simulink model "sampleModel212"  (R2021b)
settings: Solver=VariableStepAuto  StartTime=0.0  StopTime=10.0  RelTol=1e-3
undefined symbols (not defined in the file or in its folder): DiscIntNeverNeededParam, Newton, Raphson
libraries: simulink x6, slpidlib x1
settings Model: Creator=user  LastModifiedBy=user

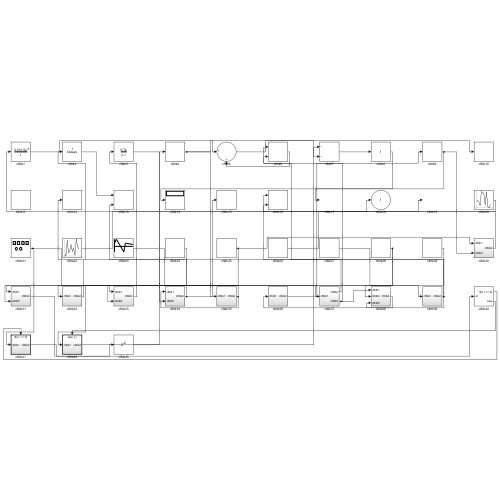
[thumbnail: Simulink's stored preview of the top-level diagram]
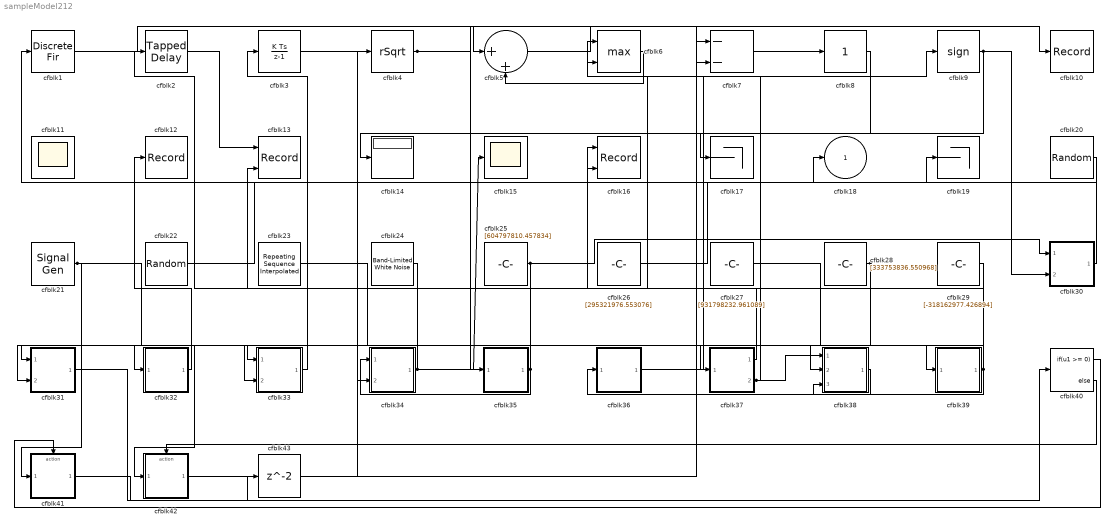
== system sampleModel212 ==
  cfblk1 : DiscreteFir  SampleTime=1
  cfblk10 : Record  FileSettingsInternal="{\"entries\":[{\"content\":{\"excelSettings\":{\"content\":{},\"type\":\"Streamout.ExcelSettings\"}},\"type\":\"Streamout.FileSettingStorage\",\"uuid\":\"9136f186-ec9e-49fd-8053-90c4ae60cd6f\"}],\"packageUris\":[\"http://schema.mathworks.com/mf0/streamout_blocks/R2020a\"],\"version\":\"1.0\"}"  SignalsInternal="{\"entries\":[{\"content\":{\"signals\":[{\"content\":{\"blockPath\":[\"sampleModel212/cfblk10\"],\"channel\":[],\"dimensions\":[1],\"domain\":\"sampleModel212/cfblk10\",\"lineColor\":\"#edb120\",\"plots\":[1],\"port\":1,\"sid\":[\"\"],\"signalID\":8232,\"signalName\":\"cfblk5\"},\"type\":\"RecordBlkView.Signal\",\"uuid\":\"3d6c6ed9-3216-4515-a2b3-ec71c8580300\"}]},\"type\":\"RecordBlkView.InputSignals\",\"uuid\":\"6f53bf0b-d229-4304-8eb9-cf2f8789923b\"}],\"packageUris\":[\"http://schema.mathworks.com/mf0/streamout_blocks/R2020a\"],\"version\":\"1.0\"}"  VisualizationBindings="{\"sparklinesplugin\":{\"info\":[{\"bindingParametersList\":[],\"subplotID\":1}]}}"
  cfblk11 : Scope
      settings: Floating=on
  cfblk12 : Record  FileSettingsInternal="{\"entries\":[{\"content\":{\"excelSettings\":{\"content\":{},\"type\":\"Streamout.ExcelSettings\"}},\"type\":\"Streamout.FileSettingStorage\",\"uuid\":\"6ba16359-3d74-4ac6-a319-7b95d1bddcf9\"}],\"packageUris\":[\"http://schema.mathworks.com/mf0/streamout_blocks/R2020a\"],\"version\":\"1.0\"}"  SignalsInternal="{\"entries\":[{\"content\":{\"signals\":[{\"content\":{\"blockPath\":[\"sampleModel212/cfblk12\"],\"channel\":[],\"dimensions\":[1],\"domain\":\"sampleModel212/cfblk12\",\"lineColor\":\"#139fff\",\"plots\":[1],\"port\":1,\"sid\":[\"\"],\"signalID\":8252,\"signalName\":\"cfblk32\"},\"type\":\"RecordBlkView.Signal\",\"uuid\":\"2d56ea30-9116-46ed-9e82-5e82888dbfa9\"}]},\"type\":\"RecordBlkView.InputSignals\",\"uuid\":\"56d7414f-cbe6-4e07-9f56-36ce9f4febc1\"}],\"packageUris\":[\"http://schema.mathworks.com/mf0/streamout_blocks/R2020a\"],\"version\":\"1.0\"}"  VisualizationBindings="{\"sparklinesplugin\":{\"info\":[{\"bindingParametersList\":[],\"subplotID\":1}]}}"
  cfblk13 : Record  FileSettingsInternal="{\"entries\":[{\"content\":{\"excelSettings\":{\"content\":{},\"type\":\"Streamout.ExcelSettings\"}},\"type\":\"Streamout.FileSettingStorage\",\"uuid\":\"0acae2d6-ee60-4856-b366-a0806cd00a70\"}],\"packageUris\":[\"http://schema.mathworks.com/mf0/streamout_blocks/R2020a\"],\"version\":\"1.0\"}"  Layout=[1 1]  SignalsInternal="{\"entries\":[{\"content\":{\"signals\":[{\"content\":{\"blockPath\":[\"sampleModel212/cfblk13\"],\"channel\":[],\"dimensions\":[1],\"domain\":\"sampleModel212/cfblk13\",\"lineColor\":\"#a2142f\",\"plots\":[1],\"port\":1,\"sid\":[\"\"],\"signalID\":8236,\"signalName\":\"cfblk2\"},\"type\":\"RecordBlkView.Signal\",\"uuid\":\"529bd515-27fc-4e1a-94ea-2d07532aa9c1\"},{\"content\":{\"blockPath\":[\"sampleModel212/cfblk13\"],\"channel\":[],\"dimensions\":[1],\"domain\":\"sampleModel212/cfblk13\",\"lineColor\":\"#139fff\",\"plots\":[1],\"port\":2,\"sid\":[\"\"],\"signalID\":8240,\"signalName\":\"cfblk39\"},\"type\":\"RecordBlkView.Signal\",\"uuid\":\"26540efe-244b-4170-a373-6d34e17a1cae\"}]},\"type\":\"RecordBlkView.InputSignals\",\"uuid\":\"31d81cea-1ae4-4f42-aa9f-f175325ecb32\"}],\"packageUris\":[\"http://schema.mathworks.com/mf0/streamout_blocks/R2020a\"],\"version\":\"1.0\"}"  VisualizationBindings="{\"xyplotplugin\":{\"info\":[{\"series\":[{\"bindingParametersList\":[{\"parameter\":\"X-Axis\",\"signalID\":8236,\"signalName\":\"cfblk2\"},{\"parameter\":\"Y-Axis\",\"signalID\":8240,\"signalName\":\"cfblk39\"}],\"seriesID\":42465}],\"subplotID\":1}]}}"  CompatibilityTag=XY
  cfblk14 : Display
  cfblk15 : Scope
  cfblk16 : Record  FileSettingsInternal="{\"entries\":[{\"content\":{\"excelSettings\":{\"content\":{},\"type\":\"Streamout.ExcelSettings\"}},\"type\":\"Streamout.FileSettingStorage\",\"uuid\":\"ca503a4a-a96d-43a1-9ebc-70d0128dd941\"}],\"packageUris\":[\"http://schema.mathworks.com/mf0/streamout_blocks/R2020a\"],\"version\":\"1.0\"}"  Layout=[1 1]  SignalsInternal="{\"entries\":[{\"content\":{\"signals\":[{\"content\":{\"blockPath\":[\"sampleModel212/cfblk16\"],\"channel\":[],\"dimensions\":[1],\"domain\":\"sampleModel212/cfblk16\",\"lineColor\":\"#a2142f\",\"plots\":[1],\"port\":1,\"sid\":[\"\"],\"signalID\":8244,\"signalName\":\"cfblk37:1\"},\"type\":\"RecordBlkView.Signal\",\"uuid\":\"e63eec24-58ba-4f65-805e-17e2aa971a90\"},{\"content\":{\"blockPath\":[\"sampleModel212/cfblk16\"],\"channel\":[],\"dimensions\":[1],\"domain\":\"sampleModel212/cfblk16\",\"lineColor\":\"#139fff\",\"plots\":[1],\"port\":2,\"sid\":[\"\"],\"signalID\":8248,\"signalName\":\"cfblk20\"},\"type\":\"RecordBlkView.Signal\",\"uuid\":\"84022ab3-d0b3-46d1-9cc4-89043ad64550\"}]},\"type\":\"RecordBlkView.InputSignals\",\"uuid\":\"213b04ee-a0f2-43b0-a9ef-411359d2bb67\"}],\"packageUris\":[\"http://schema.mathworks.com/mf0/streamout_blocks/R2020a\"],\"version\":\"1.0\"}"  VisualizationBindings="{\"xyplotplugin\":{\"info\":[{\"series\":[{\"bindingParametersList\":[{\"parameter\":\"X-Axis\",\"signalID\":8244,\"signalName\":\"cfblk37:1\"},{\"parameter\":\"Y-Axis\",\"signalID\":8248,\"signalName\":\"cfblk20\"}],\"seriesID\":43597}],\"subplotID\":1}]}}"  CompatibilityTag=XY
  cfblk17 : Terminator
  cfblk19 : Terminator
  cfblk2 : simulink/Discrete/Tapped Delay  vinit=0.0  samptime=-1  NumDelays=1  DelayOrder=Oldest  includeCurrent=off
  cfblk20 : RandomNumber  Mean=[74771.324273]  Variance=[43680.592014]  Seed=[211738287.000000]  SampleTime=0.1
  cfblk21 : SignalGenerator  WaveForm=square  Amplitude=[-349925656.261152]
  cfblk22 : UniformRandomNumber  Minimum=[-1543428115.464297]  Maximum=[1225243770.020049]  Seed=[69964703.000000]  SampleTime=0.1
  cfblk23 : simulink/Sources/Repeating Sequence Interpolated  OutValues=[224382166.710449, 496779107.925151, -364574655.609755, 227281435.577570, 132134347.634255]  TimeValues=[0 0.1 0.5 0.6 1].'  LookUpMeth=Use Input Below  tsamp=0.01  OutMin=[]  OutMax=[]  OutDataTypeStr=double  OutputDataTypeScalingMode=double  OutDataType=fixdt(0,8)  OutScaling=2^-10
  cfblk24 : simulink/Sources/Band-Limited White Noise  Cov=[1404469097.228225]  Ts=0.1  seed=[6451413531.000000]
  cfblk25 : Constant  Value=[604797810.457834]  SampleTime=1
  cfblk26 : Constant  Value=[295321976.553076]  SampleTime=1
  cfblk27 : Constant  Value=[931798232.961089]  SampleTime=1
  cfblk28 : Constant  Value=[333753836.550968]  SampleTime=1
  cfblk29 : Constant  Value=[-318162977.426894]  SampleTime=1
  cfblk3 : DiscreteIntegrator  ICPrevOutput=DiscIntNeverNeededParam  ICPrevScaledInput=DiscIntNeverNeededParam
  cfblk30 : Subsystem
  cfblk31 : Subsystem
  cfblk32 : Subsystem
  cfblk33 : Subsystem
  cfblk34 : Subsystem
  cfblk35 : Subsystem
  cfblk36 : Subsystem
  cfblk37 : Subsystem
  cfblk38 : Subsystem
  cfblk39 : Subsystem
  cfblk4 : Sqrt  Operator=rSqrt  AlgorithmType=Newton-Raphson  SaturateOnIntegerOverflow=on
  cfblk40 : If  IfExpression=u1 >= 0  SampleTime=1
  cfblk41 : Subsystem  TreatAsAtomicUnit=on
  cfblk42 : Subsystem  TreatAsAtomicUnit=on
  cfblk43 : Delay  SampleTime=1
  cfblk5 : Sum  Inputs=|++
  cfblk6 : MinMax  Function=max  Inputs=2
  cfblk7 : Sum  Inputs=--
  cfblk8 : simulink/Math Operations/Slider Gain  gain=1  low=0  high=2
  cfblk9 : Signum
  cfblk18 : Outport
  wires:
  cfblk30/1(cfblk2) -> cfblk1/1
  cfblk7/1 -> cfblk8/1
  cfblk29/1 -> cfblk32/1(cfblk1)
  cfblk2/1 -> cfblk13/1
  cfblk34/1(cfblk2) -> cfblk15/1, cfblk2/1
  cfblk32/1(cfblk2) -> cfblk12/1
  cfblk4/1 -> cfblk35/1(cfblk1), cfblk7/2
  cfblk33/1(cfblk2) -> cfblk3/1
  cfblk35/1(cfblk2) -> cfblk34/1(cfblk1), cfblk31/1(cfblk1)
  cfblk25/1 -> cfblk33/1(cfblk1), cfblk30/1(cfblk1)
  cfblk36/1(cfblk2) -> cfblk9/1
  cfblk38/1(cfblk2) -> cfblk36/1(cfblk1)
  cfblk1/1 -> cfblk5/1
  cfblk23/1 -> cfblk37/1(cfblk1)
  cfblk42/1(cfblk2) -> cfblk7/1
  cfblk39/1(cfblk2) -> cfblk13/2, cfblk38/3(cfblk5), cfblk6/1
  cfblk24/1 -> cfblk42/1(cfblk1)
  cfblk21/1 -> cfblk33/2(cfblk4), cfblk41/1(cfblk1)
  cfblk6/1 -> cfblk5/2
  cfblk8/1 -> cfblk14/1
  cfblk37/1(cfblk2) -> cfblk16/1
  cfblk27/1 -> cfblk39/1(cfblk1)
  cfblk22/1 -> cfblk18/1
  cfblk37/2(cfblk3) -> cfblk38/1(cfblk1), cfblk6/2
  cfblk20/1 -> cfblk16/2
  cfblk3/1 -> cfblk34/2(cfblk5)
  cfblk9/1 -> cfblk17/1, cfblk30/2(cfblk5)
  cfblk26/1 -> cfblk19/1
  cfblk28/1 -> cfblk38/2(cfblk4), cfblk31/2(cfblk5)
  cfblk31/1(cfblk2) -> cfblk40/1
  cfblk5/1 -> cfblk10/1
  cfblk40/1 -> cfblk41/Action
  cfblk40/2 -> cfblk42/Action
  cfblk41/1(cfblk2) -> cfblk43/1
  cfblk43/1 -> cfblk4/1

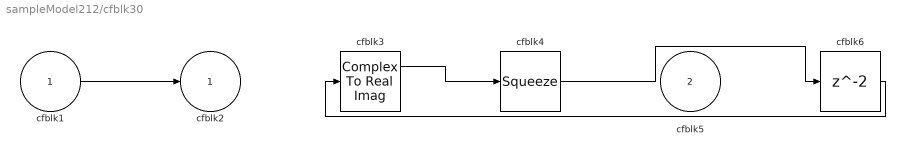
== system sampleModel212/cfblk30 ==
  cfblk1 : Inport
  cfblk5 : Inport  Port=2
  cfblk3 : ComplexToRealImag
  cfblk4 : Squeeze
  cfblk6 : Delay  SampleTime=1
  cfblk2 : Outport
  wires:
  cfblk1/1 -> cfblk2/1
  cfblk3/1 -> cfblk4/1
  cfblk4/1 -> cfblk6/1
  cfblk6/1 -> cfblk3/1

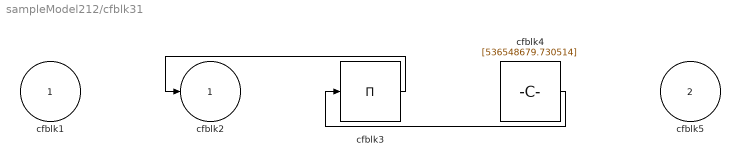
== system sampleModel212/cfblk31 ==
  cfblk1 : Inport
  cfblk5 : Inport  Port=2
  cfblk3 : Product  Inputs=*
  cfblk4 : Constant  Value=[536548679.730514]  SampleTime=1
  cfblk2 : Outport
  wires:
  cfblk3/1 -> cfblk2/1
  cfblk4/1 -> cfblk3/1

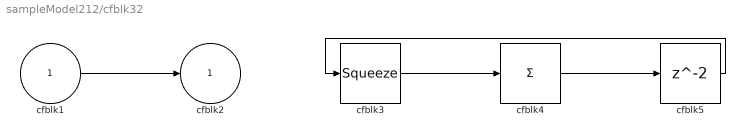
== system sampleModel212/cfblk32 ==
  cfblk1 : Inport
  cfblk3 : Squeeze
  cfblk4 : Sum  Inputs=+
  cfblk5 : Delay  SampleTime=1
  cfblk2 : Outport
  wires:
  cfblk3/1 -> cfblk4/1
  cfblk1/1 -> cfblk2/1
  cfblk4/1 -> cfblk5/1
  cfblk5/1 -> cfblk3/1

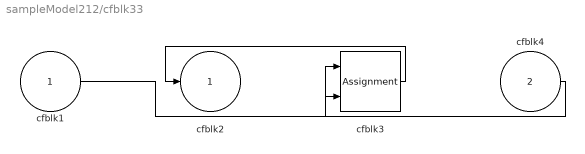
== system sampleModel212/cfblk33 ==
  cfblk1 : Inport
  cfblk4 : Inport  Port=2
  cfblk3 : Assignment  DiagnosticForDimensions=Warning  IndexOptions=Index vector (dialog)  Indices=1  OutputSizes=1
  cfblk2 : Outport
  wires:
  cfblk3/1 -> cfblk2/1
  cfblk1/1 -> cfblk3/1
  cfblk4/1 -> cfblk3/2

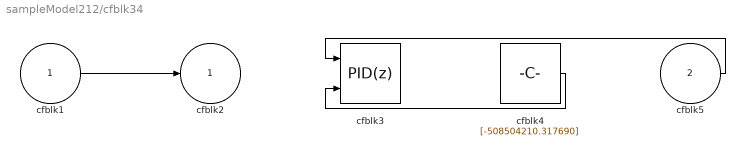
== system sampleModel212/cfblk34 ==
  cfblk1 : Inport
  cfblk5 : Inport  Port=2
  cfblk3 : slpidlib/PID Controller (2DOF)  Controller=PID  Form=Parallel  TimeDomain=Discrete-time  UseExternalTs=off  SampleTime=1  IntegratorMethod=Forward Euler  FilterMethod=Forward Euler  ControllerParametersSource=internal  P=1  I=1  D=0  UseFilter=on  N=100  b=1  c=1  TunerSelectOption=Transfer Function Based (PID Tuner App)  InitialConditionSource=internal  InitialConditionForIntegrator=0  InitialConditionForFilter=0  DifferentiatorICPrevScaledInput=0  ExternalReset=none  TrackingMode=off  Kt=1  LimitOutput=off  SatLimitsSource=internal  UpperSaturationLimit=inf  LowerSaturationLimit=-inf  LinearizeAsGain=off  AntiWindupMode=none  Kb=1  POutMin=[]  POutMax=[]  IOutMin=[]  IOutMax=[]  DOutMin=[]  DOutMax=[]  NOutMin=[]  NOutMax=[]  bOutMin=[]  bOutMax=[]  cOutMin=[]  cOutMax=[]  SumOutMin=[]  SumOutMax=[]  SaturationOutMin=[]  SaturationOutMax=[]  PParamMin=[]  PParamMax=[]  IParamMin=[]  IParamMax=[]  DParamMin=[]  DParamMax=[]  NParamMin=[]  NParamMax=[]  bParamMin=[]  bParamMax=[]  cParamMin=[]  cParamMax=[]  KbParamMin=[]  KbParamMax=[]  KtParamMin=[]  KtParamMax=[]  KbOutMin=[]  KbOutMax=[]  KtOutMin=[]  KtOutMax=[]  IntegratorOutMin=[]  IntegratorOutMax=[]  FilterOutMin=[]  FilterOutMax=[]  SumI1OutMin=[]  SumI1OutMax=[]  SumI2OutMin=[]  SumI2OutMax=[]  SumI3OutMin=[]  SumI3OutMax=[]  SumI4OutMin=[]  SumI4OutMax=[]  SumDOutMin=[]  SumDOutMax=[]  Sum1OutMin=[]  Sum1OutMax=[]  Sum2OutMin=[]  Sum2OutMax=[]  Sum3OutMin=[]  Sum3OutMax=[]  DifferentiatorOutMin=[]  DifferentiatorOutMax=[]  FilterDiffOutCoefMin=[]  FilterDiffOutCoefMax=[]  ReciprocalOutMin=[]  ReciprocalOutMax=[]  SumDenOutMin=[]  SumDenOutMax=[]  SumNumOutMin=[]  SumNumOutMax=[]  DivideOutMin=[]  DivideOutMax=[]  UdiffTsProdOutMin=[]  UdiffTsProdOutMax=[]  NTsProdOutMin=[]  NTsProdOutMax=[]  UintegralTsProdOutMin=[]  UintegralTsProdOutMax=[]  UngainTsProdOutMin=[]  UngainTsProdOutMax=[]  IntegratorContinuousStateAttributes=''  IntegratorStateMustResolveToSignalObject=off  IntegratorRTWStateStorageClass=Auto  FilterContinuousStateAttributes=''  FilterStateMustResolveToSignalObject=off  FilterRTWStateStorageClass=Auto  ParallelPVariant=InternalParameters  IdealPVariant=Disabled  IVariant=InternalParameters  DVariant=InternalParameters  bVariant=InternalParameters  cVariant=InternalParameters  IntegratorVariant=Discrete  SatVariant=Disabled  AWVariant=Passthrough  PCopyVariant=Disabled  TRVariant=Disabled  FdbkBlocksVariant=Forward  IdealPFdbkVariant=Disabled  SatFdbkVariant=Disabled  DerivativeFilterVariant=ForwardEulerFilter  NVariant=InternalParameters  NCopyVariant=Disabled  FilterICVariant=InternalICsFilter  IntegratorICVariant=InternalICs  ExternalResetVariant=Disabled  TRSumVariant=Passthrough  SumFdbkVariant=Disabled  SumVariant=Sum_PID  TsampFilterVariant=InternalTs  TsampNgainVariant=Passthrough  TsampIntegralVariant=Passthrough  ExternalSaturationOutDataTypeStr=Inherit: Same as second input
      settings: SourceProductBaseCode=SL
  cfblk4 : Constant  Value=[-508504210.317690]  SampleTime=1
  cfblk2 : Outport
  wires:
  cfblk1/1 -> cfblk2/1
  cfblk5/1 -> cfblk3/1
  cfblk4/1 -> cfblk3/2

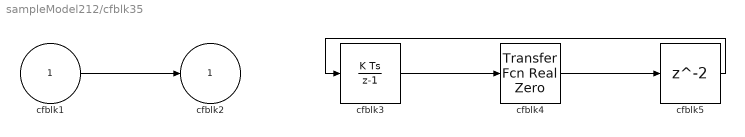
== system sampleModel212/cfblk35 ==
  cfblk1 : Inport
  cfblk3 : DiscreteIntegrator  ICPrevOutput=DiscIntNeverNeededParam  ICPrevScaledInput=DiscIntNeverNeededParam
  cfblk4 : simulink/Discrete/Transfer Fcn Real Zero  ZeroZ=0.75  ICPrevInput=0.0  DoSatur=off
      settings: SourceProductBaseCode=SL
  cfblk5 : Delay  SampleTime=1
  cfblk2 : Outport
  wires:
  cfblk1/1 -> cfblk2/1
  cfblk3/1 -> cfblk4/1
  cfblk4/1 -> cfblk5/1
  cfblk5/1 -> cfblk3/1

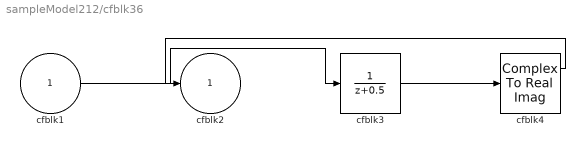
== system sampleModel212/cfblk36 ==
  cfblk1 : Inport
  cfblk3 : DiscreteTransferFcn  SampleTime=1
  cfblk4 : ComplexToRealImag
  cfblk2 : Outport
  wires:
  cfblk1/1 -> cfblk3/1
  cfblk3/1 -> cfblk4/1
  cfblk4/1 -> cfblk2/1

== system sampleModel212/cfblk37 ==
  cfblk1 : Inport
  cfblk2 : Outport
  cfblk3 : Outport  Port=2
  wires:
  cfblk1/1 -> cfblk3/1, cfblk2/1

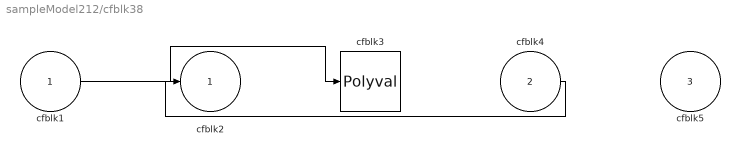
== system sampleModel212/cfblk38 ==
  cfblk1 : Inport
  cfblk4 : Inport  Port=2
  cfblk5 : Inport  Port=3
  cfblk3 : Polyval  Coefs=[ +2.081618890e-019, -1.441693666e-014, +4.719686976e-010, -8.536869453e-006, +1.621573104e-001, -8.087801117e+001 ]
  cfblk2 : Outport
  wires:
  cfblk1/1 -> cfblk3/1
  cfblk4/1 -> cfblk2/1

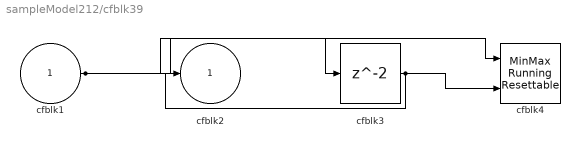
== system sampleModel212/cfblk39 ==
  cfblk1 : Inport
  cfblk3 : Delay  SampleTime=1
  cfblk4 : simulink/Math Operations/MinMax Running Resettable  Function=min  vinit=0.0
  cfblk2 : Outport
  wires:
  cfblk1/1 -> cfblk3/1, cfblk4/1
  cfblk3/1 -> cfblk2/1, cfblk4/2

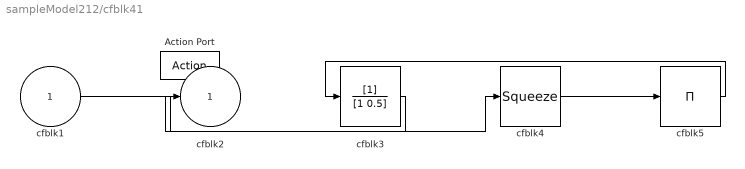
== system sampleModel212/cfblk41 ==
  cfblk1 : Inport
  Action Port : ActionPort  ActionPortLabel=if(u1 >= 0)
  cfblk3 : DiscreteFilter
  cfblk4 : Squeeze
  cfblk5 : Product  Inputs=*
  cfblk2 : Outport
  wires:
  cfblk5/1 -> cfblk3/1
  cfblk1/1 -> cfblk4/1
  cfblk4/1 -> cfblk5/1
  cfblk3/1 -> cfblk2/1

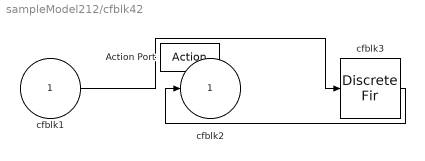
== system sampleModel212/cfblk42 ==
  cfblk1 : Inport
  Action Port : ActionPort  ActionPortLabel=else
  cfblk3 : DiscreteFir
  cfblk2 : Outport
  wires:
  cfblk3/1 -> cfblk2/1
  cfblk1/1 -> cfblk3/1
